simulink model "speed_control_of_bldc_motor_"  (R2024b)
settings: Solver=ode3  StartTime=0.0  StopTime=1  RelTol=1e-3
libraries: simulink x6, spsMosfetLib x6, spsControlledVoltageSourceLib x1, slpidlib x1, spsPermanentMagnetSynchronousMachineLib x1, sps_lib x1
settings Model: Creator=Deepak  LastModifiedBy=HP
settings SolverCC: AlgebraicLoopSolver=TrustRegion
settings DebuggingCC: UnconnectedInputMsg=warning  UnconnectedOutputMsg=warning  UnconnectedLineMsg=warning
settings ModelReferenceCC: EnableRefExpFcnMdlSchedulingChecks=on
settings SFSimCC: CustomCodeUndefinedFunction=UseInterfaceOnly
settings RTWCC: GPUComputeCapability=3.5

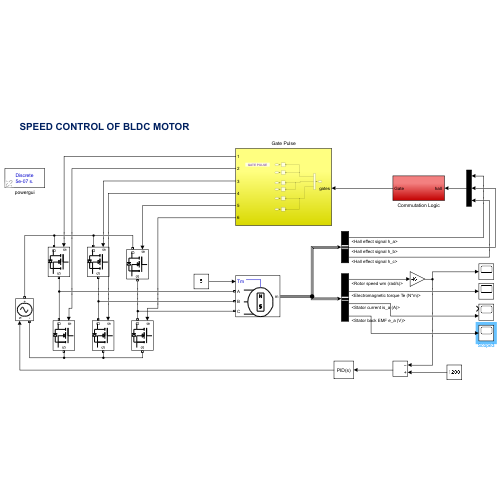
[thumbnail: Simulink's stored preview of the top-level diagram]
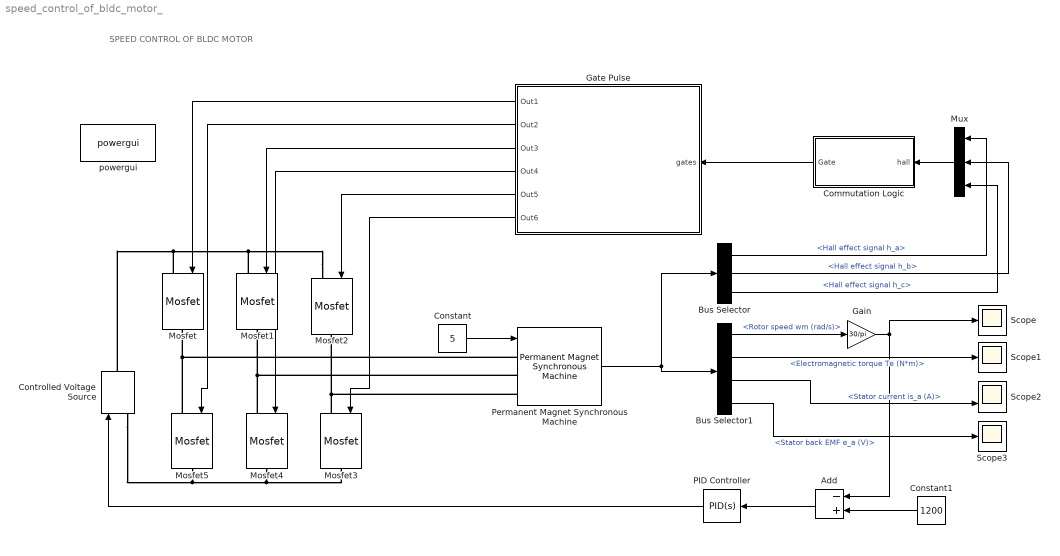
== system speed_control_of_bldc_motor_ ==
  note: SPEED CONTROL OF BLDC MOTOR
  Add : Sum  Inputs=-+
  Bus Selector : BusSelector  OutputSignals=Hall effect signal h_a,Hall effect signal h_b,Hall effect signal h_c
  Bus Selector1 : BusSelector  OutputSignals=Rotor speed wm (rad/s),Electromagnetic torque Te (N*m),Stator current is_a (A),Stator back EMF e_a (V)
  Commutation Logic : Subsystem
  Constant : Constant  Value=5
  Constant1 : Constant  Value=1200
  Controlled Voltage Source : spsControlledVoltageSourceLib/Controlled Voltage Source  Initialize=on  Source_Type=DC  Amplitude=160  Phase=0  Frequency=0  Measurements=None
  Gain : Gain  Gain=30/pi
  Gate Pulse : Subsystem
  Mosfet{,1..5} (6 alike) : spsMosfetLib/Mosfet  Ron=0.1  Lon=0  Rd=0.01  Vfd=0  IC=0  Rs=1e5  Cs=inf  Measurements=off
  Mux : Mux  Inputs=3
  PID Controller : slpidlib/PID Controller  Controller=PID  Form=Parallel  TimeDomain=Continuous-time  UseExternalTs=off  SampleTime=-1  IntegratorMethod=Forward Euler  FilterMethod=Forward Euler  ControllerParametersSource=internal  P=0.01035  I=12.777  UseKiTs=off  D=12.564  UseExternalDerivativeSource=off  N=0  UseFilter=on  TunerSelectOption=Transfer Function Based (PID Tuner App)  InitialConditionSource=internal  InitialConditionForIntegrator=0  InitialConditionForFilter=0  DifferentiatorICPrevScaledInput=0  ExternalReset=none  TrackingMode=off  Kt=1  LimitOutput=off  SatLimitsSource=internal  UpperSaturationLimit=inf  LowerSaturationLimit=-inf  LinearizeAsGain=on  AntiWindupMode=none  Kb=1  LimitIntegrator=off  UpperIntegratorSaturationLimit=inf  LowerIntegratorSaturationLimit=-inf  POutMin=[]  POutMax=[]  IOutMin=[]  IOutMax=[]  DOutMin=[]  DOutMax=[]  NOutMin=[]  NOutMax=[]  SumOutMin=[]  SumOutMax=[]  SaturationOutMin=[]  SaturationOutMax=[]  PParamMin=[]  PParamMax=[]  IParamMin=[]  IParamMax=[]  DParamMin=[]  DParamMax=[]  NParamMin=[]  NParamMax=[]  KbParamMin=[]  KbParamMax=[]  KtParamMin=[]  KtParamMax=[]  KbOutMin=[]  KbOutMax=[]  KtOutMin=[]  KtOutMax=[]  IntegratorOutMin=[]  IntegratorOutMax=[]  FilterOutMin=[]  FilterOutMax=[]  SumI1OutMin=[]  SumI1OutMax=[]  SumI2OutMin=[]  SumI2OutMax=[]  SumI3OutMin=[]  SumI3OutMax=[]  SumI4OutMin=[]  SumI4OutMax=[]  SumDOutMin=[]  SumDOutMax=[]  DifferentiatorOutMin=[]  DifferentiatorOutMax=[]  FilterDiffOutCoefMin=[]  FilterDiffOutCoefMax=[]  ReciprocalOutMin=[]  ReciprocalOutMax=[]  SumDenOutMin=[]  SumDenOutMax=[]  SumNumOutMin=[]  SumNumOutMax=[]  DivideOutMin=[]  DivideOutMax=[]  UdiffTsProdOutMin=[]  UdiffTsProdOutMax=[]  NTsProdOutMin=[]  NTsProdOutMax=[]  UintegralTsProdOutMin=[]  UintegralTsProdOutMax=[]  UngainTsProdOutMin=[]  UngainTsProdOutMax=[]  ClampingZeroOutDataTypeStr=Inherit: Inherit via back propagation  ClampingZeroOutMin=[]  ClampingZeroOutMax=[]  FilterDenConstantOutDataTypeStr=Inherit: Inherit via back propagation  FilterDenConstantOutMin=[]  FilterDenConstantOutMax=[]  PCopyOutDataTypeStr=Inherit: Inherit via back propagation  PCopyOutMin=[]  PCopyOutMax=[]  NCopyOutDataTypeStr=Inherit: Inherit via back propagation  NCopyOutMin=[]  NCopyOutMax=[]  IntegratorContinuousStateAttributes=''  IntegratorStateMustResolveToSignalObject=off  IntegratorRTWStateStorageClass=Auto  FilterContinuousStateAttributes=''  FilterStateMustResolveToSignalObject=off  FilterRTWStateStorageClass=Auto  ParallelPVariant=InternalParameters  IdealPVariant=Disabled  IVariant=InternalParameters  DVariant=InternalParameters  IntegratorVariant=Continuous  SatVariant=Disabled  AWVariant=Passthrough  PCopyVariant=Disabled  TRVariant=Disabled  FdbkBlocksVariant=Forward  IdealPFdbkVariant=Disabled  SatFdbkVariant=Disabled  DerivativeFilterVariant=ContFilter  NVariant=InternalParameters  NCopyVariant=Disabled  FilterICVariant=InternalICsFilter  IntegratorICVariant=InternalICs  ExternalResetVariant=Disabled  TRSumVariant=Passthrough  SumFdbkVariant=Disabled  SumVariant=Sum_PID  TsampFilterVariant=InternalTs  TsampNgainVariant=Passthrough  TsampIntegralVariant=Disabled_SignalSpec  ExternalSaturationOutDataTypeStr=Inherit: Same as second input  DerivativeSourceVariant=ErrorSignal  PreIntVariant=InternalPreInt
  Permanent Magnet Synchronous Machine : spsPermanentMagnetSynchronousMachineLib/Permanent Magnet Synchronous Machine  NbPhases=3  FluxDistribution=Trapezoidal  RotorType=Round  MechanicalLoad=Torque Tm  PresetModel=No  ShowDetailedParameters=on  MeasurementBus=off  Resistance=0.7  Inductance=2.7e-3  dqInductances=[8.5e-3,8.5e-3]  La=0.000395  MachineConstant=Flux linkage established by magnets (V.s)  Flux=0.1194  VoltageCst=100.0283  TorqueCst=0.9552  Flat=120  Mechanical=[0.0027 0.0004924 4 0]  PolePairs=4  InitialConditions=[0,0, 0,0]  InitialConditions5ph=[0 0 0 0 0 0]  RefAngle=90 degrees behind phase A axis (modified Park)  IterativeDiscreteModel=Trapezoidal non iterative  TsBlock=-1  TsPowergui=0
  Scope : Scope
  Scope1 : Scope
  Scope2 : Scope  NumInputPorts=2
  Scope3 : Scope
  powergui : sps_lib/powergui  Priority=1  SimulationMode=Discrete  SampleTime=50e-8  frequency=60  Iterations=50  frequencyindice=0  Pbase=100e6  ErrMax=1e-4  UnitsV=kV  UnitsW=MW  buscounter=0  FunctionMessages=off  echomessages=off  EnableUseOfTLC=off  CurrentSourceSwitches=off  DisableSnubberDevices=off  DisableRonSwitches=off  DisableVfSwitches=off  DisplayEquations=off  AutomaticDiscreteSolvers=off  SolverType=Tustin/Backward Euler (TBE)  Interpol=off  ExternalGateDelay=off  methode=off  Ts=100  x0status=blocks  SPID=on  SwTol=0  HookPort=off  NonlinearTolerance=0  nMaxIteration=15  ContinueOnMaxIteration=off  RestoreLinks=warning  ResistiveCurrentMeasurement=off  Frange=[0:2:500]  Ylog=off  Xlog=on  ShowGrid=off  save=off  variable=ZData  structure=0  ZoomFFT=off  StartTime=0.0  cycles=1  DisplayStyle=1  fundamental=60  FreqAxis=off  MaxFrequency=1000  frequencyindicesteady=1  RmsSteady=1  display=off
  wires:
  Bus Selector1/3 -> Scope2/2  "<Stator current is_a (A)>"
  Bus Selector1/4 -> Scope3/1  "<Stator back EMF e_a (V)>"
  Gate Pulse/3(Out3) -> Mosfet1/1
  Gate Pulse/5(Out5) -> Mosfet2/1
  Gate Pulse/6(Out6) -> Mosfet3/1
  Mux/1 -> Commutation Logic/1("hall ")
  Bus Selector/1 -> Mux/1  "<Hall effect signal h_a>"
  Gate Pulse/1(Out1) -> Mosfet/1
  Constant/1 -> Permanent Magnet Synchronous Machine/1
  Add/1 -> PID Controller/1
  Bus Selector1/1 -> Gain/1  "<Rotor speed wm (rad/s)>"
  PID Controller/1 -> Controlled Voltage Source/1
  Gate Pulse/4(Out4) -> Mosfet4/1
  Bus Selector1/2 -> Scope1/1  "<Electromagnetic torque Te (N*m)>"
  Constant1/1 -> Add/2
  Permanent Magnet Synchronous Machine/1 -> Bus Selector1/1, Bus Selector/1
  Gate Pulse/2(Out2) -> Mosfet5/1
  Bus Selector/3 -> Mux/3  "<Hall effect signal h_c>"
  Commutation Logic/1(Gate) -> Gate Pulse/1(gates)
  Gain/1 -> Add/1, Scope/1
  Bus Selector/2 -> Mux/2  "<Hall effect signal h_b>"
  connections:
  Mosfet2/RConn1 -- Mosfet3/LConn1 -- Permanent Magnet Synchronous Machine/LConn3
  Mosfet1/RConn1 -- Mosfet4/LConn1 -- Permanent Magnet Synchronous Machine/LConn2
  Mosfet2/LConn1 -- Mosfet/LConn1 -- Controlled Voltage Source/RConn1 -- Mosfet1/LConn1
  Mosfet/RConn1 -- Mosfet5/LConn1 -- Permanent Magnet Synchronous Machine/LConn1
  Mosfet3/RConn1 -- Mosfet5/RConn1 -- Controlled Voltage Source/LConn1 -- Mosfet4/RConn1

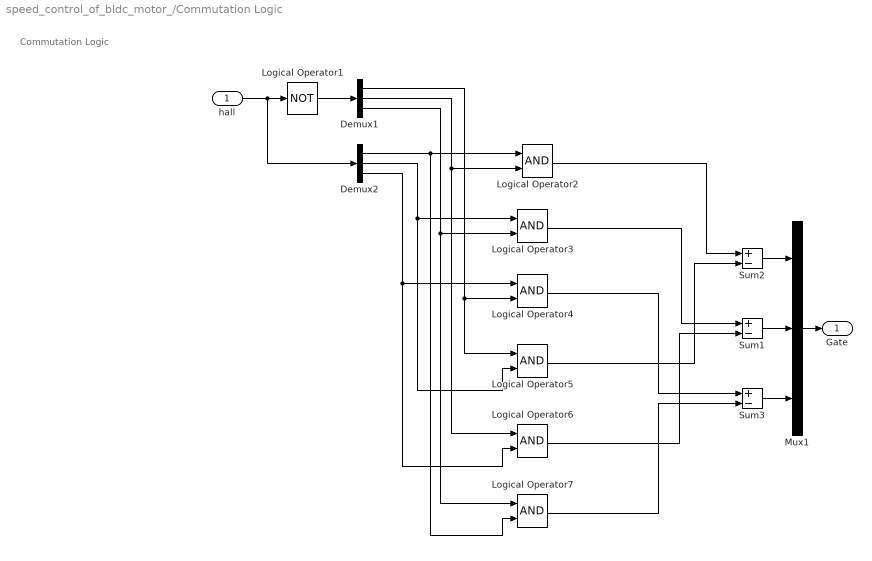
== system speed_control_of_bldc_motor_/Commutation Logic ==
  note: Commutation Logic
  "hall " : Inport
  Demux1 : Demux  Outputs=3
  Demux2 : Demux  Outputs=3
  Logical Operator1 : Logic  Operator=NOT  AllPortsSameDT=off  OutDataTypeStr=boolean
  Logical Operator{2..7} (6 alike) : Logic  AllPortsSameDT=off  OutDataTypeStr=boolean
  Mux1 : Mux  Inputs=3
  Sum1 : Sum  Inputs=+-  OutDataTypeStr=double
  Sum2 : Sum  Inputs=+-  OutDataTypeStr=double
  Sum3 : Sum  Inputs=+-  OutDataTypeStr=double
  Gate : Outport  VectorParamsAs1DForOutWhenUnconnected=off
  wires:
  Demux2/1 -> Logical Operator7/2, Logical Operator2/1
  Demux1/3 -> Logical Operator7/1, Logical Operator3/2
  Demux2/2 -> Logical Operator3/1, Logical Operator5/2
  Sum1/1 -> Mux1/2
  Logical Operator3/1 -> Sum1/1
  "hall "/1 -> Logical Operator1/1, Demux2/1
  Demux1/2 -> Logical Operator6/1, Logical Operator2/2
  Logical Operator2/1 -> Sum2/1
  Logical Operator7/1 -> Sum3/2
  Logical Operator4/1 -> Sum3/1
  Demux1/1 -> Logical Operator4/2, Logical Operator5/1
  Logical Operator6/1 -> Sum1/2
  Logical Operator5/1 -> Sum2/2
  Sum3/1 -> Mux1/3
  Logical Operator1/1 -> Demux1/1
  Mux1/1 -> Gate/1
  Sum2/1 -> Mux1/1
  Demux2/3 -> Logical Operator4/1, Logical Operator6/2

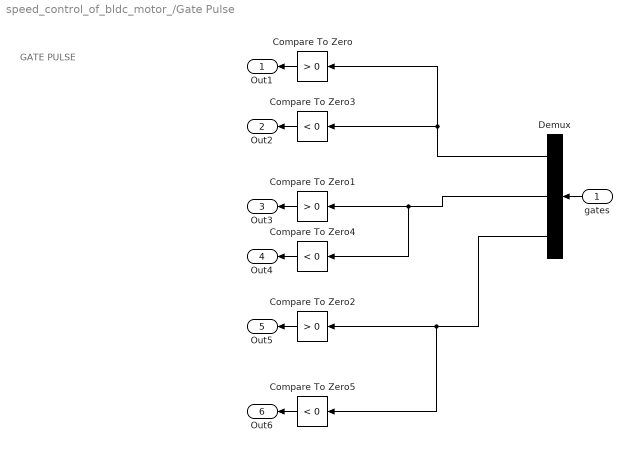
== system speed_control_of_bldc_motor_/Gate Pulse ==
  note: GATE PULSE
  gates : Inport
  Compare To Zero : simulink/Logic and Bit Operations/Compare To Zero  relop=>  OutDataTypeStr=boolean
  Compare To Zero1 : simulink/Logic and Bit Operations/Compare To Zero  relop=>  OutDataTypeStr=boolean
  Compare To Zero2 : simulink/Logic and Bit Operations/Compare To Zero  relop=>  OutDataTypeStr=boolean
  Compare To Zero3 : simulink/Logic and Bit Operations/Compare To Zero  relop=<  OutDataTypeStr=boolean
  Compare To Zero4 : simulink/Logic and Bit Operations/Compare To Zero  relop=<  OutDataTypeStr=boolean
  Compare To Zero5 : simulink/Logic and Bit Operations/Compare To Zero  relop=<  OutDataTypeStr=boolean
  Demux : Demux  Outputs=3
  Out1 : Outport  VectorParamsAs1DForOutWhenUnconnected=off
  Out2 : Outport  Port=2  VectorParamsAs1DForOutWhenUnconnected=off
  Out3 : Outport  Port=3  VectorParamsAs1DForOutWhenUnconnected=off
  Out4 : Outport  Port=4  VectorParamsAs1DForOutWhenUnconnected=off
  Out5 : Outport  Port=5  VectorParamsAs1DForOutWhenUnconnected=off
  Out6 : Outport  Port=6  VectorParamsAs1DForOutWhenUnconnected=off
  wires:
  Compare To Zero1/1 -> Out3/1
  Demux/2 -> Compare To Zero4/1, Compare To Zero1/1
  Compare To Zero3/1 -> Out2/1
  Demux/3 -> Compare To Zero5/1, Compare To Zero2/1
  Compare To Zero2/1 -> Out5/1
  Demux/1 -> Compare To Zero3/1, Compare To Zero/1
  Compare To Zero4/1 -> Out4/1
  Compare To Zero5/1 -> Out6/1
  Compare To Zero/1 -> Out1/1
  gates/1 -> Demux/1
